simulink model "lvwenjing"  (R2019a)
settings: Solver=VariableStepAuto  StartTime=0.0  StopTime=10.0  RelTol=1e-3
libraries: dsparch4 x2
settings Model: Creator=Sherlock Holmes  LastModifiedBy=Sherlock Holmes

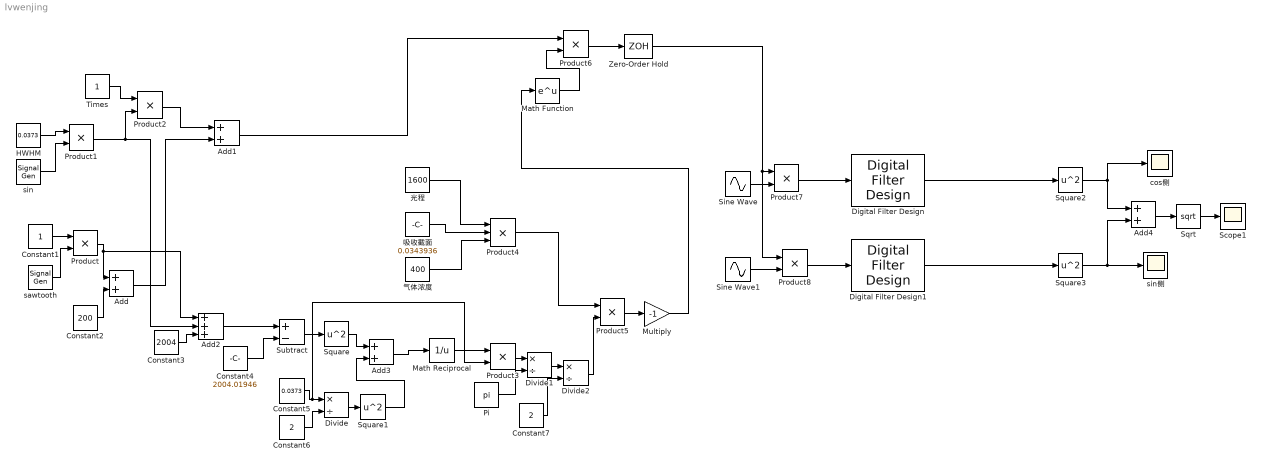
== system lvwenjing ==
  Add{,1,3..4} (4 alike) : Sum
  Add2 : Sum  Inputs=+++
  Constant1 : Constant
  Constant2 : Constant  Value=200
  Constant3 : Constant  Value=2004
  Constant4 : Constant  Value=2004.01946
  Constant5 : Constant  Value=0.0373
  Constant6 : Constant  Value=2
  Constant7 : Constant  Value=2
  Digital Filter Design : dsparch4/Digital Filter Design  mwdsp_browser_bugfix_var=off
  Digital Filter Design1 : dsparch4/Digital Filter Design  mwdsp_browser_bugfix_var=off
  Divide : Product  Inputs=*/
  Divide1 : Product  Inputs=*/
  Divide2 : Product  Inputs=*/
  HWHM : Constant  Value=0.0373
  Math Function : Math  SaturateOnIntegerOverflow=on
  Math Reciprocal : Math  Operator=reciprocal  SaturateOnIntegerOverflow=on
  Multiply : Gain  Gain=-1
  Pi : Constant  Value=pi  OutDataTypeStr=Inherit: Inherit via back propagation
  Product{,1..3,5..8} (8 alike) : Product
  Product4 : Product  Inputs=3
  Scope1 : Scope
  Sine Wave : Sin  Frequency=40000  Phase=pi/2  SampleTime=0
  Sine Wave1 : Sin  Frequency=40000  SampleTime=0
  Sqrt : Sqrt  SaturateOnIntegerOverflow=on
  Square{,1..3} (4 alike) : Math  Operator=square  SaturateOnIntegerOverflow=on
  Subtract : Sum  Inputs=+-
  Times : Constant
  Zero-Order Hold : ZeroOrderHold  SampleTime=-1
  cos侧 : Scope
  sawtooth : SignalGenerator  WaveForm=sawtooth  Frequency=2
  sin : SignalGenerator  Frequency=20000
  sin侧 : Scope
  光程 : Constant  Value=1600
  吸收截面 : Constant  Value=0.0343936
  气体浓度 : Constant  Value=400
  wires:
  sawtooth/1 -> Product/2
  Constant1/1 -> Product/1
  Constant2/1 -> Add/2
  Product/1 -> Add/1, Add2/1
  Add/1 -> Add1/2
  HWHM/1 -> Product1/1
  sin/1 -> Product1/2
  Times/1 -> Product2/1
  Product1/1 -> Add2/2, Product2/2
  Product2/1 -> Add1/1
  Constant3/1 -> Add2/3
  Add2/1 -> Subtract/1
  Constant4/1 -> Subtract/2
  Subtract/1 -> Square/1
  Square/1 -> Add3/1
  Constant5/1 -> Product3/2, Divide/1
  Constant6/1 -> Divide/2
  Divide/1 -> Square1/1
  Square1/1 -> Add3/2
  Add3/1 -> Math Reciprocal/1
  Math Reciprocal/1 -> Product3/1
  Product3/1 -> Divide1/1
  Pi/1 -> Divide1/2
  Divide1/1 -> Divide2/1
  Constant7/1 -> Divide2/2
  光程/1 -> Product4/1
  吸收截面/1 -> Product4/2
  气体浓度/1 -> Product4/3
  Divide2/1 -> Product5/2
  Product4/1 -> Product5/1
  Product5/1 -> Multiply/1
  Multiply/1 -> Math Function/1
  Math Function/1 -> Product6/2
  Add1/1 -> Product6/1
  Sine Wave/1 -> Product7/2
  Sine Wave1/1 -> Product8/2
  Product8/1 -> Digital Filter Design1/1
  Product7/1 -> Digital Filter Design/1
  Square2/1 -> cos侧/1, Add4/1
  Square3/1 -> sin侧/1, Add4/2
  Add4/1 -> Sqrt/1
  Sqrt/1 -> Scope1/1
  Digital Filter Design/1 -> Square2/1
  Digital Filter Design1/1 -> Square3/1
  Product6/1 -> Zero-Order Hold/1
  Zero-Order Hold/1 -> Product8/1, Product7/1
